simulink model "xpcUEIDualasync"  (Simulink 6.0)
settings: Solver=FixedStepDiscrete  StartTime=0.0  StopTime=inf  FixedStep=.001  RelTol=1e-3
undefined symbols (not defined in the file or in its folder): MF, MFS, PD2
libraries: xpclib x8, dspsigattribs x2
settings Model: Creator=gweast  LastModifiedBy=ekbas  ExtModeArmWhenConnect=off  BufferReuse=off  ProdHWDeviceType=Specified  xpc_rtwmakecfg_data=_xpcuei_
settings DataIOCC: SignalLoggingName=sigsOut
settings OptimizationCC: InlineInvariantSignals=off  OptimizeBlockIOStorage=off  BufferReuse=off  EnforceIntegerDowncast=off  FoldNonRolledExpr=off  LocalBlockOutputs=off  MultiInstanced=off
settings FormatCC: IgnoreBidirectionalLines=off
settings HardwareCC: ProdHWDeviceType=Specified
settings RTWCC: SystemTargetFile=xpctarget.tlc  TemplateMakefile=xpc_default_tmf  ProcessScript=xpctarget_make_rtw_hook
settings CodeAppCC: SimulinkBlockComments=off
settings xpcTargetCC: TargetFcnLib=iso_c_tmw.mat

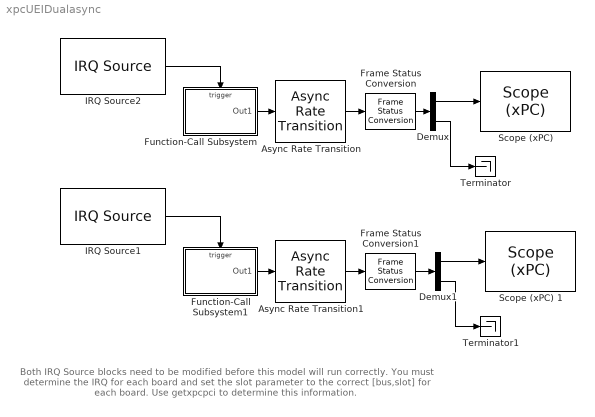
== system xpcUEIDualasync ==
  note: Both IRQ Source blocks need to be modified before this model
      | will run correctly.  You must determine the IRQ for each board
      | and set the slot parameter to the correct [bus,slot] for each
      | board.  Use getxpcpci to determine this information.
  Async Rate Transition : xpclib/Asynchronous Event/Async Rate Transition  sample_time=-1
  Async Rate Transition1 : xpclib/Asynchronous Event/Async Rate Transition  sample_time=-1
  Demux : Demux  Outputs=[5 -1]
  Demux1 : Demux  Outputs=[5 -1]
  Frame Status Conversion : dspsigattribs/Frame Status Conversion  growRefPort=off  outframe=Sample-based
  Frame Status Conversion1 : dspsigattribs/Frame Status Conversion  growRefPort=off  outframe=Sample-based
  Function-Call Subsystem : Subsystem  TreatAsAtomicUnit=on
  Function-Call Subsystem1 : Subsystem  TreatAsAtomicUnit=on
  IRQ Source1 : xpclib/Asynchronous Event/IRQ Source  irqNo=9  preempt=on  b_type=UEI_MFx  slot=-1
  IRQ Source2 : xpclib/Asynchronous Event/IRQ Source  irqNo=10  preempt=on  b_type=UEI_MFx  slot=-1
  "Scope (xPC) " : xpclib/Misc./Scope (xPC)   scopeno=1  scopetype=Target  autostart=on  viewmode=Graphical redraw  formatstr='%15.6f'  grid=on  ylimits=[0,0]  nosamples=500  noprepostsamples=0  interleave=1  triggermode=FreeRun  triggersignal=1  triggerlevel=0.0  triggerslope=Either  triggerscope=1  triggersample=0  filename=data.dat  mode=Lazy  writesize=512  autorestart=off
  Scope (xPC) 1 : xpclib/Misc./Scope (xPC)   scopeno=2  scopetype=Target  autostart=on  viewmode=Graphical redraw  formatstr='%15.6f'  grid=on  ylimits=[0,0]  nosamples=500  noprepostsamples=0  interleave=1  triggermode=FreeRun  triggersignal=1  triggerlevel=0.0  triggerslope=Either  triggerscope=1  triggersample=0  filename=data.dat  mode=Lazy  writesize=512  autorestart=off
  Terminator : Terminator
  Terminator1 : Terminator
  wires:
  IRQ Source2/1 -> Function-Call Subsystem/Trigger
  Function-Call Subsystem/1(Out1) -> Async Rate Transition/1
  Frame Status Conversion/1 -> Demux/1
  Demux/1 -> "Scope (xPC) "/1
  Demux/2 -> Terminator/1
  Async Rate Transition/1 -> Frame Status Conversion/1
  IRQ Source1/1 -> Function-Call Subsystem1/Trigger
  Function-Call Subsystem1/1(Out1) -> Async Rate Transition1/1
  Async Rate Transition1/1 -> Frame Status Conversion1/1
  Frame Status Conversion1/1 -> Demux1/1
  Demux1/1 -> Scope (xPC) 1/1
  Demux1/2 -> Terminator1/1

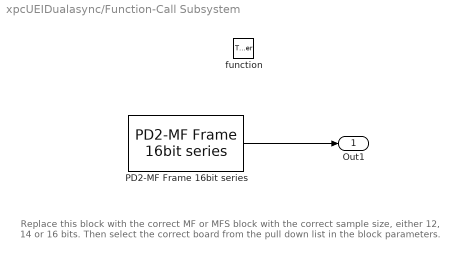
== system xpcUEIDualasync/Function-Call Subsystem ==
  note: Replace this block with the correct MF or MFS block with the correct
      | sample size, either 12, 14 or 16 bits.  Then select the correct board
      | from the pull down list in the block parameters.
  function : TriggerPort  TriggerType=function-call
  "PD2-MF Frame 16bit series " : xpclib/A//D Frame/UEI/PD2-MF Frame 16bit series   boardtypein=PD2-MF-16-333/16H  channel=[1]  gain=[1]  mux=[0]  range=+- 10 Volts  sediff=Single Ended  framesize=32  outfmt=Frame (Signal Processing blockset needed)  clsource=Internal  scantime=-1  frametime=0.001  sampletime=on  slave=off  freq=-1  burst=32  pcislot=-1
  Out1 : Outport
  wires:
  "PD2-MF Frame 16bit series "/1 -> Out1/1

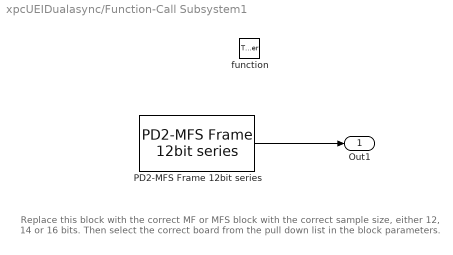
== system xpcUEIDualasync/Function-Call Subsystem1 ==
  note: Replace this block with the correct MF or MFS block with the correct
      | sample size, either 12, 14 or 16 bits.  Then select the correct board
      | from the pull down list in the block parameters.
  function : TriggerPort  TriggerType=function-call
  "PD2-MFS Frame 12bit series " : xpclib/A//D Frame/UEI/PD2-MFS Frame 12bit series   boardtypein=PD2-MFS-4-1M/12  channel=[1]  gain=[1]  mux=[0]  range=+- 10 Volts  framesize=32  outfmt=Frame (Signal Processing blockset needed)  clsource=Internal  scantime=-1  frametime=0.001  sampletime=on  slave=off  freq=-1  burst=32  pcislot=-1
  Out1 : Outport
  wires:
  "PD2-MFS Frame 12bit series "/1 -> Out1/1
